simulink model "DFIG_and_Big_Generator"  (R2023a)
settings: Solver=ode45  StartTime=0.0  StopTime=10  RelTol=1e-2  EnableMultiTasking=on
PreLoadFcn:
  | assignin('base','Ts',[2e-6])
undefined symbols (not defined in the file): D1, Delta, DiscIntNeverNeededParam, find_system, Ion, level, Lithium, Ts
libraries: powerlib_extras x83, spsThreePhaseVIMeasurementLib x16, spsThreePhaseBreakerLib x16, simulink_extras x12, spsThreePhaseTransformerTwoWindingsLib x8, spsPLL3phLib x5, spsPowerPLLDrivenPositiveSequenceLib x5, spsUniversalBridgeLib x5, spsThreePhaseSeriesRLCLoadLib x5, spsThreePhaseSeriesRLCBranchLib x4, spsGroundLib x3, spsFundamentalPLLDrivenLib x2
(part 6 of 6)

== system DFIG_and_Big_Generator/DFIG Wind Turbine/Control/Measurement and Transformation/Discrete 3-phase PLL-Driven Positive-Sequence Active & Reactive Power/Discrete 3-phase PLL-Driven Positive-Sequence Fundamental Value/Discrete Variable Frequency Mean value1/Correction subsystem ==
  N : Inport
  F : Inport  Port=2
  In : Inport  Port=3
  Gain1 : Gain  Gain=0.5  SaturateOnIntegerOverflow=on  OutDataTypeStr=Inherit: Same as input  ParamDataTypeStr=Inherit: Same as input
  Product2 : Product  Inputs=*/  InputSameDT=on  SaturateOnIntegerOverflow=on  OutDataTypeStr=Inherit: Same as first input
  Product4 : Product  Inputs=**  InputSameDT=on  SaturateOnIntegerOverflow=on  OutDataTypeStr=Inherit: Same as first input
  Product5 : Product  Inputs=**  InputSameDT=on  SaturateOnIntegerOverflow=on  OutDataTypeStr=Inherit: Same as first input
  Sum1 : Sum  Inputs=+-  InputSameDT=on  SaturateOnIntegerOverflow=on  OutDataTypeStr=Inherit: Same as first input
  Sum4 : Sum  InputSameDT=on  SaturateOnIntegerOverflow=on  OutDataTypeStr=Inherit: Same as first input
  Sum5 : Sum  Inputs=+-  InputSameDT=on  SaturateOnIntegerOverflow=on  OutDataTypeStr=Inherit: Same as first input
  Unit Delay : UnitDelay  SampleTime=Ts  HasFrameUpgradeWarning=on
  Out : Outport
  wires:
  Unit Delay/1 -> Sum1/2
  N/1 -> Sum5/1, Product2/2
  F/1 -> Sum5/2
  Sum5/1 -> Product2/1, Product5/1
  Product2/1 -> Product4/1
  In/1 -> Sum1/1, Unit Delay/1, Sum4/2
  Sum1/1 -> Product5/2
  Product5/1 -> Gain1/1
  Gain1/1 -> Sum4/1
  Sum4/1 -> Product4/2
  Product4/1 -> Out/1

== system DFIG_and_Big_Generator/DFIG Wind Turbine/Control/Measurement and Transformation/Discrete 3-phase PLL-Driven Positive-Sequence Active & Reactive Power/Discrete 3-phase PLL-Driven Positive-Sequence Fundamental Value/Discrete Variable Frequency Mean value1/Discrete Variable Transport Delay ==
  In : Inport
  D : Inport  Port=2
  "S-Function " : S-Function  FunctionName=discreteVariableTransportDelay  Parameters=MaxDelay,Ts,InitialValue  SFunctionDeploymentMode=off  EnableBusSupport=off
  Out : Outport
  wires:
  "S-Function "/1 -> Out/1
  In/1 -> "S-Function "/1
  D/1 -> "S-Function "/2

== system DFIG_and_Big_Generator/DFIG Wind Turbine/Control/Measurement and Transformation/Discrete 3-phase PLL-Driven Positive-Sequence Active & Reactive Power/Discrete 3-phase PLL-Driven Positive-Sequence Fundamental Value/Discrete Variable Frequency Mean value2/Correction subsystem ==
  N : Inport
  F : Inport  Port=2
  In : Inport  Port=3
  Gain1 : Gain  Gain=0.5  SaturateOnIntegerOverflow=on  OutDataTypeStr=Inherit: Same as input  ParamDataTypeStr=Inherit: Same as input
  Product2 : Product  Inputs=*/  InputSameDT=on  SaturateOnIntegerOverflow=on  OutDataTypeStr=Inherit: Same as first input
  Product4 : Product  Inputs=**  InputSameDT=on  SaturateOnIntegerOverflow=on  OutDataTypeStr=Inherit: Same as first input
  Product5 : Product  Inputs=**  InputSameDT=on  SaturateOnIntegerOverflow=on  OutDataTypeStr=Inherit: Same as first input
  Sum1 : Sum  Inputs=+-  InputSameDT=on  SaturateOnIntegerOverflow=on  OutDataTypeStr=Inherit: Same as first input
  Sum4 : Sum  InputSameDT=on  SaturateOnIntegerOverflow=on  OutDataTypeStr=Inherit: Same as first input
  Sum5 : Sum  Inputs=+-  InputSameDT=on  SaturateOnIntegerOverflow=on  OutDataTypeStr=Inherit: Same as first input
  Unit Delay : UnitDelay  SampleTime=Ts  HasFrameUpgradeWarning=on
  Out : Outport
  wires:
  Product4/1 -> Out/1
  Sum4/1 -> Product4/2
  Gain1/1 -> Sum4/1
  Product5/1 -> Gain1/1
  Sum1/1 -> Product5/2
  In/1 -> Sum4/2, Unit Delay/1, Sum1/1
  Product2/1 -> Product4/1
  Sum5/1 -> Product5/1, Product2/1
  F/1 -> Sum5/2
  N/1 -> Product2/2, Sum5/1
  Unit Delay/1 -> Sum1/2

== system DFIG_and_Big_Generator/DFIG Wind Turbine/Control/Measurement and Transformation/Discrete 3-phase PLL-Driven Positive-Sequence Active & Reactive Power/Discrete 3-phase PLL-Driven Positive-Sequence Fundamental Value/Discrete Variable Frequency Mean value2/Discrete Variable Transport Delay ==
  In : Inport
  D : Inport  Port=2
  "S-Function " : S-Function  FunctionName=discreteVariableTransportDelay  Parameters=MaxDelay,Ts,InitialValue  SFunctionDeploymentMode=off  EnableBusSupport=off
  Out : Outport
  wires:
  D/1 -> "S-Function "/2
  In/1 -> "S-Function "/1
  "S-Function "/1 -> Out/1

== system DFIG_and_Big_Generator/DFIG Wind Turbine/Control/Measurement and Transformation/Discrete 3-phase PLL-Driven Positive-Sequence Active & Reactive Power/Discrete 3-phase PLL-Driven Positive-Sequence Fundamental Value2/Discrete Variable Frequency Mean value1/Correction subsystem ==
  N : Inport
  F : Inport  Port=2
  In : Inport  Port=3
  Gain1 : Gain  Gain=0.5  SaturateOnIntegerOverflow=on  OutDataTypeStr=Inherit: Same as input  ParamDataTypeStr=Inherit: Same as input
  Product2 : Product  Inputs=*/  InputSameDT=on  SaturateOnIntegerOverflow=on  OutDataTypeStr=Inherit: Same as first input
  Product4 : Product  Inputs=**  InputSameDT=on  SaturateOnIntegerOverflow=on  OutDataTypeStr=Inherit: Same as first input
  Product5 : Product  Inputs=**  InputSameDT=on  SaturateOnIntegerOverflow=on  OutDataTypeStr=Inherit: Same as first input
  Sum1 : Sum  Inputs=+-  InputSameDT=on  SaturateOnIntegerOverflow=on  OutDataTypeStr=Inherit: Same as first input
  Sum4 : Sum  InputSameDT=on  SaturateOnIntegerOverflow=on  OutDataTypeStr=Inherit: Same as first input
  Sum5 : Sum  Inputs=+-  InputSameDT=on  SaturateOnIntegerOverflow=on  OutDataTypeStr=Inherit: Same as first input
  Unit Delay : UnitDelay  SampleTime=Ts  HasFrameUpgradeWarning=on
  Out : Outport
  wires:
  Product4/1 -> Out/1
  Sum4/1 -> Product4/2
  Gain1/1 -> Sum4/1
  Product5/1 -> Gain1/1
  Sum1/1 -> Product5/2
  In/1 -> Sum4/2, Unit Delay/1, Sum1/1
  Product2/1 -> Product4/1
  Sum5/1 -> Product5/1, Product2/1
  F/1 -> Sum5/2
  N/1 -> Product2/2, Sum5/1
  Unit Delay/1 -> Sum1/2

== system DFIG_and_Big_Generator/DFIG Wind Turbine/Control/Measurement and Transformation/Discrete 3-phase PLL-Driven Positive-Sequence Active & Reactive Power/Discrete 3-phase PLL-Driven Positive-Sequence Fundamental Value2/Discrete Variable Frequency Mean value1/Discrete Variable Transport Delay ==
  In : Inport
  D : Inport  Port=2
  "S-Function " : S-Function  FunctionName=discreteVariableTransportDelay  Parameters=MaxDelay,Ts,InitialValue  SFunctionDeploymentMode=off  EnableBusSupport=off
  Out : Outport
  wires:
  D/1 -> "S-Function "/2
  In/1 -> "S-Function "/1
  "S-Function "/1 -> Out/1

== system DFIG_and_Big_Generator/DFIG Wind Turbine/Control/Measurement and Transformation/Discrete 3-phase PLL-Driven Positive-Sequence Active & Reactive Power/Discrete 3-phase PLL-Driven Positive-Sequence Fundamental Value2/Discrete Variable Frequency Mean value2/Correction subsystem ==
  N : Inport
  F : Inport  Port=2
  In : Inport  Port=3
  Gain1 : Gain  Gain=0.5  SaturateOnIntegerOverflow=on  OutDataTypeStr=Inherit: Same as input  ParamDataTypeStr=Inherit: Same as input
  Product2 : Product  Inputs=*/  InputSameDT=on  SaturateOnIntegerOverflow=on  OutDataTypeStr=Inherit: Same as first input
  Product4 : Product  Inputs=**  InputSameDT=on  SaturateOnIntegerOverflow=on  OutDataTypeStr=Inherit: Same as first input
  Product5 : Product  Inputs=**  InputSameDT=on  SaturateOnIntegerOverflow=on  OutDataTypeStr=Inherit: Same as first input
  Sum1 : Sum  Inputs=+-  InputSameDT=on  SaturateOnIntegerOverflow=on  OutDataTypeStr=Inherit: Same as first input
  Sum4 : Sum  InputSameDT=on  SaturateOnIntegerOverflow=on  OutDataTypeStr=Inherit: Same as first input
  Sum5 : Sum  Inputs=+-  InputSameDT=on  SaturateOnIntegerOverflow=on  OutDataTypeStr=Inherit: Same as first input
  Unit Delay : UnitDelay  SampleTime=Ts  HasFrameUpgradeWarning=on
  Out : Outport
  wires:
  Unit Delay/1 -> Sum1/2
  N/1 -> Sum5/1, Product2/2
  F/1 -> Sum5/2
  Sum5/1 -> Product2/1, Product5/1
  Product2/1 -> Product4/1
  In/1 -> Sum1/1, Unit Delay/1, Sum4/2
  Sum1/1 -> Product5/2
  Product5/1 -> Gain1/1
  Gain1/1 -> Sum4/1
  Sum4/1 -> Product4/2
  Product4/1 -> Out/1

== system DFIG_and_Big_Generator/DFIG Wind Turbine/Control/Measurement and Transformation/Discrete 3-phase PLL-Driven Positive-Sequence Active & Reactive Power/Discrete 3-phase PLL-Driven Positive-Sequence Fundamental Value2/Discrete Variable Frequency Mean value2/Discrete Variable Transport Delay ==
  In : Inport
  D : Inport  Port=2
  "S-Function " : S-Function  FunctionName=discreteVariableTransportDelay  Parameters=MaxDelay,Ts,InitialValue  SFunctionDeploymentMode=off  EnableBusSupport=off
  Out : Outport
  wires:
  "S-Function "/1 -> Out/1
  In/1 -> "S-Function "/1
  D/1 -> "S-Function "/2

== system DFIG_and_Big_Generator/DFIG Wind Turbine1/Control/Measurement and Transformation/Discrete 3-phase PLL-Driven Positive-Sequence Active & Reactive Power/Discrete 3-phase PLL-Driven Positive-Sequence Fundamental Value/Discrete Variable Frequency Mean value1/Correction subsystem ==
  N : Inport
  F : Inport  Port=2
  In : Inport  Port=3
  Gain1 : Gain  Gain=0.5  SaturateOnIntegerOverflow=on  OutDataTypeStr=Inherit: Same as input  ParamDataTypeStr=Inherit: Same as input
  Product2 : Product  Inputs=*/  InputSameDT=on  SaturateOnIntegerOverflow=on  OutDataTypeStr=Inherit: Same as first input
  Product4 : Product  Inputs=**  InputSameDT=on  SaturateOnIntegerOverflow=on  OutDataTypeStr=Inherit: Same as first input
  Product5 : Product  Inputs=**  InputSameDT=on  SaturateOnIntegerOverflow=on  OutDataTypeStr=Inherit: Same as first input
  Sum1 : Sum  Inputs=+-  InputSameDT=on  SaturateOnIntegerOverflow=on  OutDataTypeStr=Inherit: Same as first input
  Sum4 : Sum  InputSameDT=on  SaturateOnIntegerOverflow=on  OutDataTypeStr=Inherit: Same as first input
  Sum5 : Sum  Inputs=+-  InputSameDT=on  SaturateOnIntegerOverflow=on  OutDataTypeStr=Inherit: Same as first input
  Unit Delay : UnitDelay  SampleTime=Ts  HasFrameUpgradeWarning=on
  Out : Outport
  wires:
  Product4/1 -> Out/1
  Sum4/1 -> Product4/2
  Gain1/1 -> Sum4/1
  Product5/1 -> Gain1/1
  Sum1/1 -> Product5/2
  In/1 -> Sum4/2, Unit Delay/1, Sum1/1
  Product2/1 -> Product4/1
  Sum5/1 -> Product5/1, Product2/1
  F/1 -> Sum5/2
  N/1 -> Product2/2, Sum5/1
  Unit Delay/1 -> Sum1/2

== system DFIG_and_Big_Generator/DFIG Wind Turbine1/Control/Measurement and Transformation/Discrete 3-phase PLL-Driven Positive-Sequence Active & Reactive Power/Discrete 3-phase PLL-Driven Positive-Sequence Fundamental Value/Discrete Variable Frequency Mean value1/Discrete Variable Transport Delay ==
  In : Inport
  D : Inport  Port=2
  "S-Function " : S-Function  FunctionName=discreteVariableTransportDelay  Parameters=MaxDelay,Ts,InitialValue  SFunctionDeploymentMode=off  EnableBusSupport=off
  Out : Outport
  wires:
  D/1 -> "S-Function "/2
  In/1 -> "S-Function "/1
  "S-Function "/1 -> Out/1

== system DFIG_and_Big_Generator/DFIG Wind Turbine1/Control/Measurement and Transformation/Discrete 3-phase PLL-Driven Positive-Sequence Active & Reactive Power/Discrete 3-phase PLL-Driven Positive-Sequence Fundamental Value/Discrete Variable Frequency Mean value2/Correction subsystem ==
  N : Inport
  F : Inport  Port=2
  In : Inport  Port=3
  Gain1 : Gain  Gain=0.5  SaturateOnIntegerOverflow=on  OutDataTypeStr=Inherit: Same as input  ParamDataTypeStr=Inherit: Same as input
  Product2 : Product  Inputs=*/  InputSameDT=on  SaturateOnIntegerOverflow=on  OutDataTypeStr=Inherit: Same as first input
  Product4 : Product  Inputs=**  InputSameDT=on  SaturateOnIntegerOverflow=on  OutDataTypeStr=Inherit: Same as first input
  Product5 : Product  Inputs=**  InputSameDT=on  SaturateOnIntegerOverflow=on  OutDataTypeStr=Inherit: Same as first input
  Sum1 : Sum  Inputs=+-  InputSameDT=on  SaturateOnIntegerOverflow=on  OutDataTypeStr=Inherit: Same as first input
  Sum4 : Sum  InputSameDT=on  SaturateOnIntegerOverflow=on  OutDataTypeStr=Inherit: Same as first input
  Sum5 : Sum  Inputs=+-  InputSameDT=on  SaturateOnIntegerOverflow=on  OutDataTypeStr=Inherit: Same as first input
  Unit Delay : UnitDelay  SampleTime=Ts  HasFrameUpgradeWarning=on
  Out : Outport
  wires:
  Unit Delay/1 -> Sum1/2
  N/1 -> Sum5/1, Product2/2
  F/1 -> Sum5/2
  Sum5/1 -> Product2/1, Product5/1
  Product2/1 -> Product4/1
  In/1 -> Sum1/1, Unit Delay/1, Sum4/2
  Sum1/1 -> Product5/2
  Product5/1 -> Gain1/1
  Gain1/1 -> Sum4/1
  Sum4/1 -> Product4/2
  Product4/1 -> Out/1

== system DFIG_and_Big_Generator/DFIG Wind Turbine1/Control/Measurement and Transformation/Discrete 3-phase PLL-Driven Positive-Sequence Active & Reactive Power/Discrete 3-phase PLL-Driven Positive-Sequence Fundamental Value/Discrete Variable Frequency Mean value2/Discrete Variable Transport Delay ==
  In : Inport
  D : Inport  Port=2
  "S-Function " : S-Function  FunctionName=discreteVariableTransportDelay  Parameters=MaxDelay,Ts,InitialValue  SFunctionDeploymentMode=off  EnableBusSupport=off
  Out : Outport
  wires:
  "S-Function "/1 -> Out/1
  In/1 -> "S-Function "/1
  D/1 -> "S-Function "/2

== system DFIG_and_Big_Generator/DFIG Wind Turbine1/Control/Measurement and Transformation/Discrete 3-phase PLL-Driven Positive-Sequence Active & Reactive Power/Discrete 3-phase PLL-Driven Positive-Sequence Fundamental Value2/Discrete Variable Frequency Mean value1/Correction subsystem ==
  N : Inport
  F : Inport  Port=2
  In : Inport  Port=3
  Gain1 : Gain  Gain=0.5  SaturateOnIntegerOverflow=on  OutDataTypeStr=Inherit: Same as input  ParamDataTypeStr=Inherit: Same as input
  Product2 : Product  Inputs=*/  InputSameDT=on  SaturateOnIntegerOverflow=on  OutDataTypeStr=Inherit: Same as first input
  Product4 : Product  Inputs=**  InputSameDT=on  SaturateOnIntegerOverflow=on  OutDataTypeStr=Inherit: Same as first input
  Product5 : Product  Inputs=**  InputSameDT=on  SaturateOnIntegerOverflow=on  OutDataTypeStr=Inherit: Same as first input
  Sum1 : Sum  Inputs=+-  InputSameDT=on  SaturateOnIntegerOverflow=on  OutDataTypeStr=Inherit: Same as first input
  Sum4 : Sum  InputSameDT=on  SaturateOnIntegerOverflow=on  OutDataTypeStr=Inherit: Same as first input
  Sum5 : Sum  Inputs=+-  InputSameDT=on  SaturateOnIntegerOverflow=on  OutDataTypeStr=Inherit: Same as first input
  Unit Delay : UnitDelay  SampleTime=Ts  HasFrameUpgradeWarning=on
  Out : Outport
  wires:
  Unit Delay/1 -> Sum1/2
  N/1 -> Sum5/1, Product2/2
  F/1 -> Sum5/2
  Sum5/1 -> Product2/1, Product5/1
  Product2/1 -> Product4/1
  In/1 -> Sum1/1, Unit Delay/1, Sum4/2
  Sum1/1 -> Product5/2
  Product5/1 -> Gain1/1
  Gain1/1 -> Sum4/1
  Sum4/1 -> Product4/2
  Product4/1 -> Out/1

== system DFIG_and_Big_Generator/DFIG Wind Turbine1/Control/Measurement and Transformation/Discrete 3-phase PLL-Driven Positive-Sequence Active & Reactive Power/Discrete 3-phase PLL-Driven Positive-Sequence Fundamental Value2/Discrete Variable Frequency Mean value1/Discrete Variable Transport Delay ==
  In : Inport
  D : Inport  Port=2
  "S-Function " : S-Function  FunctionName=discreteVariableTransportDelay  Parameters=MaxDelay,Ts,InitialValue  SFunctionDeploymentMode=off  EnableBusSupport=off
  Out : Outport
  wires:
  "S-Function "/1 -> Out/1
  In/1 -> "S-Function "/1
  D/1 -> "S-Function "/2

== system DFIG_and_Big_Generator/DFIG Wind Turbine1/Control/Measurement and Transformation/Discrete 3-phase PLL-Driven Positive-Sequence Active & Reactive Power/Discrete 3-phase PLL-Driven Positive-Sequence Fundamental Value2/Discrete Variable Frequency Mean value2/Correction subsystem ==
  N : Inport
  F : Inport  Port=2
  In : Inport  Port=3
  Gain1 : Gain  Gain=0.5  SaturateOnIntegerOverflow=on  OutDataTypeStr=Inherit: Same as input  ParamDataTypeStr=Inherit: Same as input
  Product2 : Product  Inputs=*/  InputSameDT=on  SaturateOnIntegerOverflow=on  OutDataTypeStr=Inherit: Same as first input
  Product4 : Product  Inputs=**  InputSameDT=on  SaturateOnIntegerOverflow=on  OutDataTypeStr=Inherit: Same as first input
  Product5 : Product  Inputs=**  InputSameDT=on  SaturateOnIntegerOverflow=on  OutDataTypeStr=Inherit: Same as first input
  Sum1 : Sum  Inputs=+-  InputSameDT=on  SaturateOnIntegerOverflow=on  OutDataTypeStr=Inherit: Same as first input
  Sum4 : Sum  InputSameDT=on  SaturateOnIntegerOverflow=on  OutDataTypeStr=Inherit: Same as first input
  Sum5 : Sum  Inputs=+-  InputSameDT=on  SaturateOnIntegerOverflow=on  OutDataTypeStr=Inherit: Same as first input
  Unit Delay : UnitDelay  SampleTime=Ts  HasFrameUpgradeWarning=on
  Out : Outport
  wires:
  Product4/1 -> Out/1
  Sum4/1 -> Product4/2
  Gain1/1 -> Sum4/1
  Product5/1 -> Gain1/1
  Sum1/1 -> Product5/2
  In/1 -> Sum4/2, Unit Delay/1, Sum1/1
  Product2/1 -> Product4/1
  Sum5/1 -> Product5/1, Product2/1
  F/1 -> Sum5/2
  N/1 -> Product2/2, Sum5/1
  Unit Delay/1 -> Sum1/2

== system DFIG_and_Big_Generator/DFIG Wind Turbine1/Control/Measurement and Transformation/Discrete 3-phase PLL-Driven Positive-Sequence Active & Reactive Power/Discrete 3-phase PLL-Driven Positive-Sequence Fundamental Value2/Discrete Variable Frequency Mean value2/Discrete Variable Transport Delay ==
  In : Inport
  D : Inport  Port=2
  "S-Function " : S-Function  FunctionName=discreteVariableTransportDelay  Parameters=MaxDelay,Ts,InitialValue  SFunctionDeploymentMode=off  EnableBusSupport=off
  Out : Outport
  wires:
  D/1 -> "S-Function "/2
  In/1 -> "S-Function "/1
  "S-Function "/1 -> Out/1
